simulink model "Optimized_Architecture"  (R2015b)
settings: Solver=FixedStepDiscrete  SolverMode=SingleTasking  StartTime=0.0  StopTime=1000e-6  RelTol=1e-3
libraries: shlslibv1 x282
(part 1 of 2)
settings Model: synDspstartup=OK  Creator=smohan21  LastModifiedBy=smohan21
settings DataIOCC: SaveOutput=off  SignalLogging=off  SaveTime=off
settings OptimizationCC: DefaultParameterBehavior=Inlined
settings DebuggingCC: AlgebraicLoopMsg=error  InheritedTsInSrcMsg=none

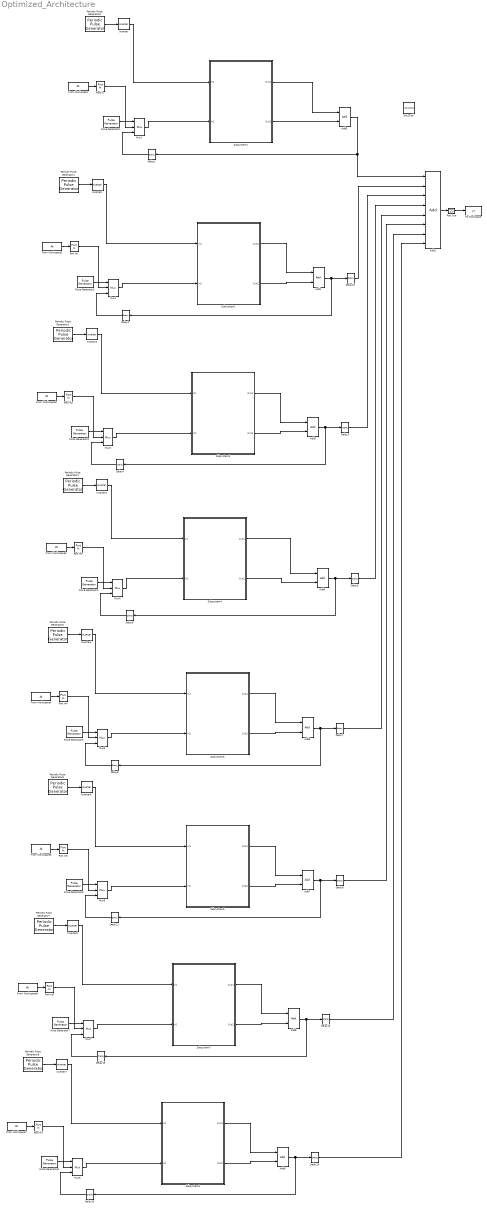
== system Optimized_Architecture ==
  Add{1,3..9} (8 alike) : shlslibv1/Math Functions/Add  syn_add_opr=++  syn_out_f=Specify  syn_out_wl=10  syn_out_fl=0  syn_out_dt=unsigned  syn_out_sat=off  syn_out_rnd=Floor (Truncate)  synBlockType=primitive  synLatency=0  synBlockId=96  syn_sum_of_rows=off  syn_inh_port=off  syn_inh_st=on  syn_inh_stf=1  syn_en_pipe=off  syn_pipe_stg=10  syn_flow_ctrl=off
  Add2 : shlslibv1/Math Functions/Add  syn_add_opr=++++++++  syn_out_f=Specify  syn_out_wl=10  syn_out_fl=0  syn_out_dt=unsigned  syn_out_sat=off  syn_out_rnd=Floor (Truncate)  synBlockType=primitive  synLatency=0  synBlockId=96  syn_sum_of_rows=off  syn_inh_port=off  syn_inh_st=on  syn_inh_stf=1  syn_en_pipe=off  syn_pipe_stg=10  syn_flow_ctrl=off
  Delay{1..2,4,6,8,11,13,15} (8 alike) : shlslibv1/Memories/Delay  syn_delay_val=32  synBlockType=primitive  synLatency=32  synBlockId=104
  Delay10 : shlslibv1/Memories/Delay  syn_delay_val=30  synBlockType=primitive  synLatency=30  synBlockId=104
  Delay12 : shlslibv1/Memories/Delay  syn_delay_val=180  synBlockType=primitive  synLatency=180  synBlockId=104
  Delay14 : shlslibv1/Memories/Delay  syn_delay_val=210  synBlockType=primitive  synLatency=210  synBlockId=104
  Delay3 : shlslibv1/Memories/Delay  syn_delay_val=60  synBlockType=primitive  synLatency=60  synBlockId=104
  Delay5 : shlslibv1/Memories/Delay  syn_delay_val=90  synBlockType=primitive  synLatency=90  synBlockId=104
  Delay7 : shlslibv1/Memories/Delay  syn_delay_val=120  synBlockType=primitive  synLatency=120  synBlockId=104
  Delay9 : shlslibv1/Memories/Delay  syn_delay_val=150  synBlockType=primitive  synLatency=150  synBlockId=104
  From Workspace{,1..7} (8 alike) : FromWorkspace  VariableName=At
  Inverter{,1..7} (8 alike) : shlslibv1/Math Functions/Inverter  syn_out_f=Automatic  syn_out_wl=16  syn_out_fl=8  syn_out_dt=signed  synBlockType=primitive  synLatency=0  synBlockId=10
  Mux{1..8} (8 alike) : shlslibv1/Signal Operations/Mux  syn_in_nb=2  syn_out_f=Specify  syn_out_wl=10  syn_out_fl=0  syn_out_dt=unsigned  syn_en_se=off  synBlockType=primitive  synLatency=0  synBlockId=16
  Periodic Pulse Generator{1..8} (8 alike) : shlslibv1/Sources/Periodic Pulse  Generator  syn_period_type=Constant  syn_period=312  syn_pw_type=Constant  syn_pw=31  syn_pd_type=Constant  syn_pd=0  syn_en_port=off  syn_st=1/1e6  synBlockType=custom  synLatency=0
  Port In{,1..7} (8 alike) : shlslibv1/Ports & Subsystems/Port In  syn_out_wl=10  syn_out_fl=0  syn_out_dt=signed  syn_out_st=-1  syn_capture=off  syn_register=on  syn_out_sat=off  syn_out_rnd=on  synBlockType=port  synLatency=1  synBlockId=0
  Port Out : shlslibv1/Ports & Subsystems/Port Out  syn_capture=off  syn_register=on  synBlockType=port  synLatency=1  synBlockId=1
  Pulse Generator{1..8} (8 alike) : shlslibv1/Sources/Pulse Generator  syn_siggentype=Step (0 to 1)  syn_usectl=off  syn_trigedge=rising  syn_triginit=low  syn_stpdel=31  syn_impwidth=1  syn_impdel=1  syn_st=1/1e6  synBlockType=custom  synLatency=0
  SHLSTool : shlslibv1/SHLSTool  synBlockType=tool  syn_dsp_mode=FPGA
  Subsystem1 : Subsystem
  Subsystem2 : Subsystem
  Subsystem3 : Subsystem
  Subsystem4 : Subsystem
  Subsystem5 : Subsystem
  Subsystem6 : Subsystem
  Subsystem7 : Subsystem
  Subsystem8 : Subsystem
  To Workspace : ToWorkspace  VariableName=yt  SaveFormat=Structure With Time  SampleTime=-1
  wires:
  From Workspace/1 -> Port In/1
  Add5/1 -> Delay1/1, Add2/1
  Periodic Pulse Generator3/1 -> Inverter/1
  Pulse Generator1/1 -> Mux2/1
  Port In/1 -> Mux2/2
  Delay1/1 -> Mux2/3
  Add1/1 -> Delay2/1, Delay10/1
  Delay10/1 -> Add2/2
  Add2/1 -> Port Out/1
  Inverter/1 -> Subsystem2/1(In1)
  Mux2/1 -> Subsystem2/2(In2)
  Subsystem2/1(Out1) -> Add5/1
  Subsystem2/2(Out2) -> Add5/2
  From Workspace1/1 -> Port In1/1
  Periodic Pulse Generator1/1 -> Inverter1/1
  Pulse Generator2/1 -> Mux1/1
  Port In1/1 -> Mux1/2
  Delay2/1 -> Mux1/3
  Inverter1/1 -> Subsystem1/1(In1)
  Mux1/1 -> Subsystem1/2(In2)
  Subsystem1/1(Out1) -> Add1/1
  Subsystem1/2(Out2) -> Add1/2
  Add3/1 -> Delay4/1, Delay3/1
  From Workspace2/1 -> Port In2/1
  Periodic Pulse Generator2/1 -> Inverter2/1
  Pulse Generator3/1 -> Mux3/1
  Port In2/1 -> Mux3/2
  Delay4/1 -> Mux3/3
  Inverter2/1 -> Subsystem3/1(In1)
  Mux3/1 -> Subsystem3/2(In2)
  Subsystem3/1(Out1) -> Add3/1
  Subsystem3/2(Out2) -> Add3/2
  Add4/1 -> Delay6/1, Delay5/1
  From Workspace3/1 -> Port In3/1
  Periodic Pulse Generator4/1 -> Inverter3/1
  Pulse Generator4/1 -> Mux4/1
  Port In3/1 -> Mux4/2
  Delay6/1 -> Mux4/3
  Inverter3/1 -> Subsystem4/1(In1)
  Mux4/1 -> Subsystem4/2(In2)
  Subsystem4/1(Out1) -> Add4/1
  Subsystem4/2(Out2) -> Add4/2
  Add6/1 -> Delay8/1, Delay7/1
  From Workspace4/1 -> Port In4/1
  Periodic Pulse Generator5/1 -> Inverter4/1
  Pulse Generator5/1 -> Mux5/1
  Port In4/1 -> Mux5/2
  Delay8/1 -> Mux5/3
  Inverter4/1 -> Subsystem5/1(In1)
  Mux5/1 -> Subsystem5/2(In2)
  Subsystem5/1(Out1) -> Add6/1
  Subsystem5/2(Out2) -> Add6/2
  Add7/1 -> Delay11/1, Delay9/1
  From Workspace5/1 -> Port In5/1
  Periodic Pulse Generator6/1 -> Inverter5/1
  Pulse Generator6/1 -> Mux6/1
  Port In5/1 -> Mux6/2
  Delay11/1 -> Mux6/3
  Inverter5/1 -> Subsystem6/1(In1)
  Mux6/1 -> Subsystem6/2(In2)
  Subsystem6/1(Out1) -> Add7/1
  Subsystem6/2(Out2) -> Add7/2
  Add8/1 -> Delay13/1, Delay12/1
  From Workspace6/1 -> Port In6/1
  Periodic Pulse Generator7/1 -> Inverter6/1
  Pulse Generator7/1 -> Mux7/1
  Port In6/1 -> Mux7/2
  Delay13/1 -> Mux7/3
  Inverter6/1 -> Subsystem7/1(In1)
  Mux7/1 -> Subsystem7/2(In2)
  Subsystem7/1(Out1) -> Add8/1
  Subsystem7/2(Out2) -> Add8/2
  Add9/1 -> Delay15/1, Delay14/1
  From Workspace7/1 -> Port In7/1
  Periodic Pulse Generator8/1 -> Inverter7/1
  Pulse Generator8/1 -> Mux8/1
  Port In7/1 -> Mux8/2
  Delay15/1 -> Mux8/3
  Inverter7/1 -> Subsystem8/1(In1)
  Mux8/1 -> Subsystem8/2(In2)
  Subsystem8/1(Out1) -> Add9/1
  Subsystem8/2(Out2) -> Add9/2
  Delay3/1 -> Add2/3
  Delay5/1 -> Add2/4
  Delay7/1 -> Add2/5
  Delay9/1 -> Add2/6
  Delay12/1 -> Add2/7
  Delay14/1 -> Add2/8
  Port Out/1 -> To Workspace/1

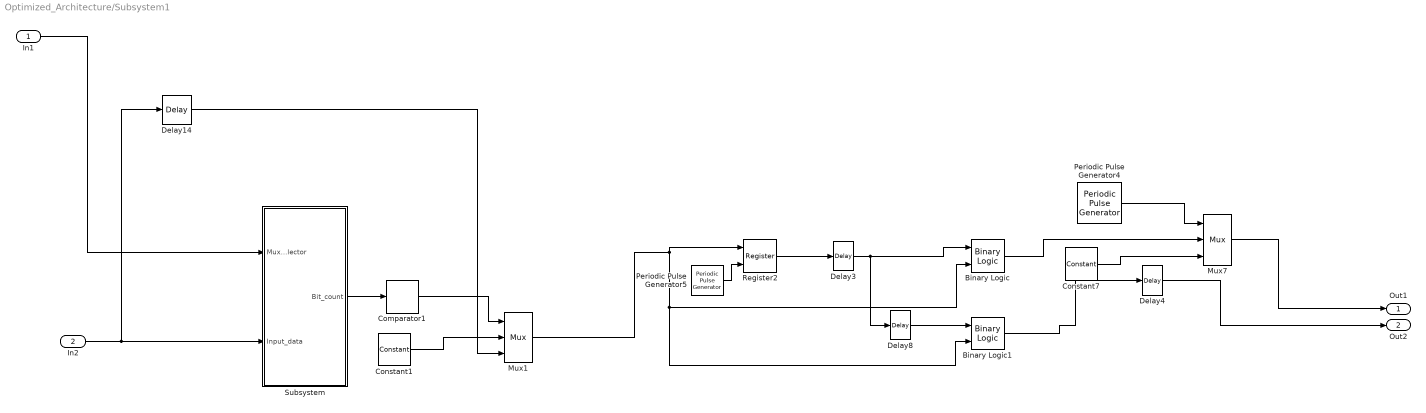
== system Optimized_Architecture/Subsystem1 ==
  In1 : Inport
  In2 : Inport  Port=2
  Binary Logic : shlslibv1/Math Functions/Binary Logic  syn_binlog_exp=a&b  synBlockType=primitive  synLatency=0  synBlockId=13
  Binary Logic1 : shlslibv1/Math Functions/Binary Logic  syn_binlog_exp=a&b  synBlockType=primitive  synLatency=0  synBlockId=13
  Comparator1 : shlslibv1/Math Functions/Comparator  syn_comp_opr=a>=b  syn_comp_const=on  syn_comp_val=2  syn_en_se=off  synBlockType=primitive  synLatency=0  synBlockId=14
  Constant1 : shlslibv1/Sources/Constant  syn_cst_val=0  syn_cst_format=Automatic  syn_cst_wl=1  syn_cst_fl=0  syn_cst_dt=unsigned  syn_cst_rnd=on  syn_cst_st=-1  synBlockType=primitive  synLatency=0  synBlockId=15
  Constant7 : shlslibv1/Sources/Constant  syn_cst_val=0  syn_cst_format=Automatic  syn_cst_wl=1  syn_cst_fl=0  syn_cst_dt=unsigned  syn_cst_rnd=on  syn_cst_st=-1  synBlockType=primitive  synLatency=0  synBlockId=15
  Delay14 : shlslibv1/Memories/Delay  syn_delay_val=270  synBlockType=primitive  synLatency=270  synBlockId=104
  Delay3 : shlslibv1/Memories/Delay  syn_delay_val=9  synBlockType=primitive  synLatency=9  synBlockId=104
  Delay4 : shlslibv1/Memories/Delay  syn_delay_val=10  synBlockType=primitive  synLatency=10  synBlockId=104
  Delay8 : shlslibv1/Memories/Delay  syn_delay_val=10  synBlockType=primitive  synLatency=10  synBlockId=104
  Mux1 : shlslibv1/Signal Operations/Mux  syn_in_nb=2  syn_out_f=Specify  syn_out_wl=10  syn_out_fl=0  syn_out_dt=unsigned  syn_en_se=off  synBlockType=primitive  synLatency=0  synBlockId=16
  Mux7 : shlslibv1/Signal Operations/Mux  syn_in_nb=2  syn_out_f=Specify  syn_out_wl=10  syn_out_fl=0  syn_out_dt=unsigned  syn_en_se=off  synBlockType=primitive  synLatency=0  synBlockId=16
  Periodic Pulse Generator4 : shlslibv1/Sources/Periodic Pulse  Generator  syn_period_type=Constant  syn_period=312  syn_pw_type=Constant  syn_pw=31  syn_pd_type=Constant  syn_pd=0  syn_en_port=off  syn_st=1/1e6  synBlockType=custom  synLatency=0
  Periodic Pulse Generator5 : shlslibv1/Sources/Periodic Pulse  Generator  syn_period_type=Constant  syn_period=270  syn_pw_type=Constant  syn_pw=1  syn_pd_type=Constant  syn_pd=0  syn_en_port=off  syn_st=1/1e6  synBlockType=custom  synLatency=0
  Register2 : shlslibv1/Memories/Register  syn_delay_val=1  syn_rst_val=All zeros  syn_rst_vec=5  syn_rst_port=on  syn_en_port=off  synBlockType=custom  synLatency=1
  Subsystem : Subsystem
  Out1 : Outport
  Out2 : Outport  Port=2
  wires:
  In1/1 -> Subsystem/1(Mux_selector)
  Mux7/1 -> Out1/1
  Mux1/1 -> Register2/1, Binary Logic/2, Binary Logic1/2
  Subsystem/1(Bit_count) -> Comparator1/1
  Constant1/1 -> Mux1/2
  Delay14/1 -> Mux1/3
  Delay3/1 -> Binary Logic/1, Delay8/1
  Binary Logic1/1 -> Delay4/1
  Comparator1/1 -> Mux1/1
  Periodic Pulse Generator4/1 -> Mux7/1
  In2/1 -> Delay14/1, Subsystem/2(Input_data)
  Register2/1 -> Delay3/1
  Delay8/1 -> Binary Logic1/1
  Constant7/1 -> Mux7/3
  Periodic Pulse Generator5/1 -> Register2/2
  Binary Logic/1 -> Mux7/2
  Delay4/1 -> Out2/1

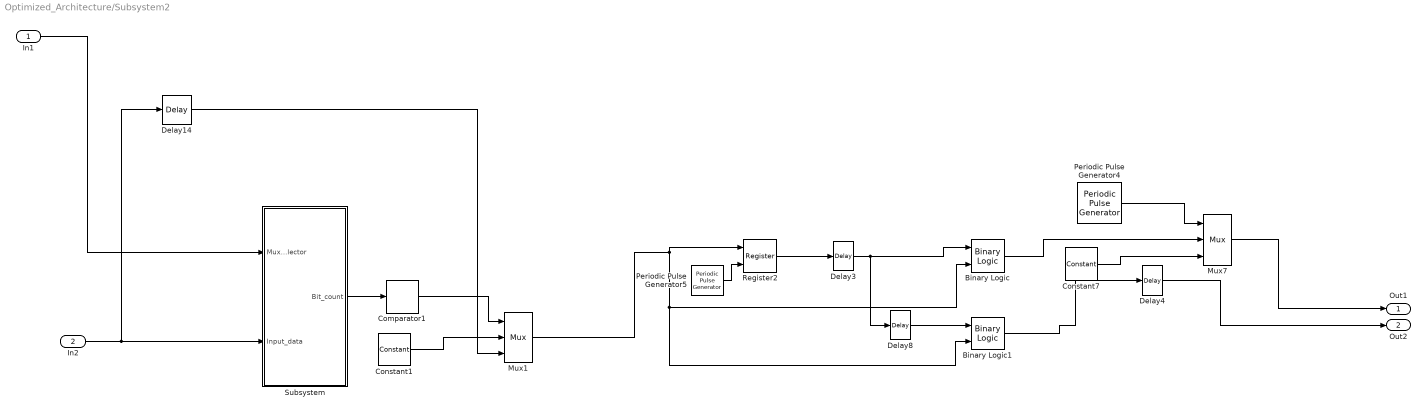
== system Optimized_Architecture/Subsystem2 ==
  In1 : Inport
  In2 : Inport  Port=2
  Binary Logic : shlslibv1/Math Functions/Binary Logic  syn_binlog_exp=a&b  synBlockType=primitive  synLatency=0  synBlockId=13
  Binary Logic1 : shlslibv1/Math Functions/Binary Logic  syn_binlog_exp=a&b  synBlockType=primitive  synLatency=0  synBlockId=13
  Comparator1 : shlslibv1/Math Functions/Comparator  syn_comp_opr=a>=b  syn_comp_const=on  syn_comp_val=2  syn_en_se=off  synBlockType=primitive  synLatency=0  synBlockId=14
  Constant1 : shlslibv1/Sources/Constant  syn_cst_val=0  syn_cst_format=Automatic  syn_cst_wl=1  syn_cst_fl=0  syn_cst_dt=unsigned  syn_cst_rnd=on  syn_cst_st=-1  synBlockType=primitive  synLatency=0  synBlockId=15
  Constant7 : shlslibv1/Sources/Constant  syn_cst_val=0  syn_cst_format=Automatic  syn_cst_wl=1  syn_cst_fl=0  syn_cst_dt=unsigned  syn_cst_rnd=on  syn_cst_st=-1  synBlockType=primitive  synLatency=0  synBlockId=15
  Delay14 : shlslibv1/Memories/Delay  syn_delay_val=270  synBlockType=primitive  synLatency=270  synBlockId=104
  Delay3 : shlslibv1/Memories/Delay  syn_delay_val=9  synBlockType=primitive  synLatency=9  synBlockId=104
  Delay4 : shlslibv1/Memories/Delay  syn_delay_val=10  synBlockType=primitive  synLatency=10  synBlockId=104
  Delay8 : shlslibv1/Memories/Delay  syn_delay_val=10  synBlockType=primitive  synLatency=10  synBlockId=104
  Mux1 : shlslibv1/Signal Operations/Mux  syn_in_nb=2  syn_out_f=Specify  syn_out_wl=10  syn_out_fl=0  syn_out_dt=unsigned  syn_en_se=off  synBlockType=primitive  synLatency=0  synBlockId=16
  Mux7 : shlslibv1/Signal Operations/Mux  syn_in_nb=2  syn_out_f=Specify  syn_out_wl=10  syn_out_fl=0  syn_out_dt=unsigned  syn_en_se=off  synBlockType=primitive  synLatency=0  synBlockId=16
  Periodic Pulse Generator4 : shlslibv1/Sources/Periodic Pulse  Generator  syn_period_type=Constant  syn_period=312  syn_pw_type=Constant  syn_pw=31  syn_pd_type=Constant  syn_pd=0  syn_en_port=off  syn_st=1/1e6  synBlockType=custom  synLatency=0
  Periodic Pulse Generator5 : shlslibv1/Sources/Periodic Pulse  Generator  syn_period_type=Constant  syn_period=270  syn_pw_type=Constant  syn_pw=1  syn_pd_type=Constant  syn_pd=0  syn_en_port=off  syn_st=1/1e6  synBlockType=custom  synLatency=0
  Register2 : shlslibv1/Memories/Register  syn_delay_val=1  syn_rst_val=All zeros  syn_rst_vec=5  syn_rst_port=on  syn_en_port=off  synBlockType=custom  synLatency=1
  Subsystem : Subsystem
  Out1 : Outport
  Out2 : Outport  Port=2
  wires:
  In1/1 -> Subsystem/1(Mux_selector)
  Mux7/1 -> Out1/1
  Mux1/1 -> Register2/1, Binary Logic/2, Binary Logic1/2
  Subsystem/1(Bit_count) -> Comparator1/1
  Constant1/1 -> Mux1/2
  Delay14/1 -> Mux1/3
  Delay3/1 -> Binary Logic/1, Delay8/1
  Binary Logic1/1 -> Delay4/1
  Comparator1/1 -> Mux1/1
  Periodic Pulse Generator4/1 -> Mux7/1
  In2/1 -> Delay14/1, Subsystem/2(Input_data)
  Register2/1 -> Delay3/1
  Delay8/1 -> Binary Logic1/1
  Constant7/1 -> Mux7/3
  Periodic Pulse Generator5/1 -> Register2/2
  Binary Logic/1 -> Mux7/2
  Delay4/1 -> Out2/1

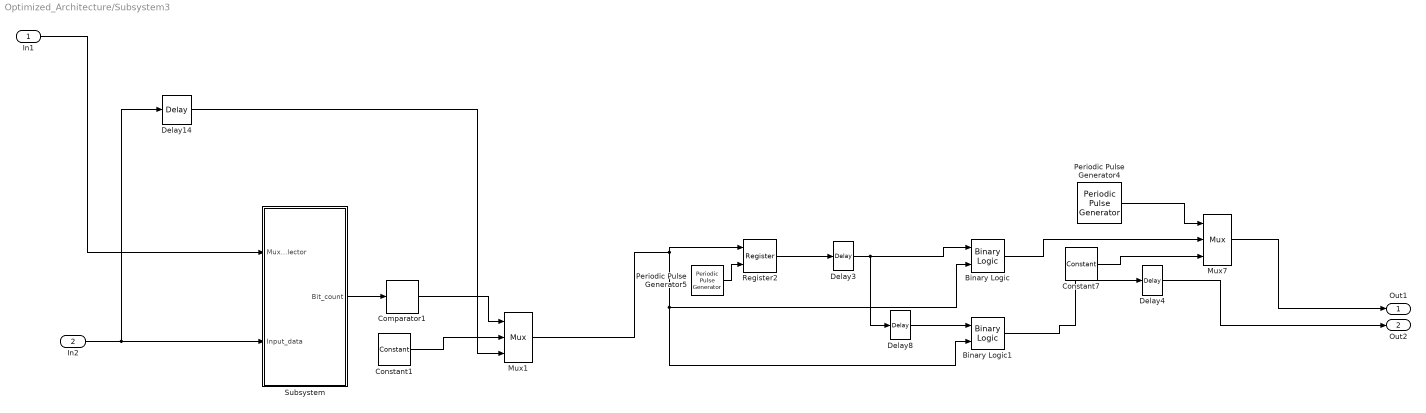
== system Optimized_Architecture/Subsystem3 ==
  In1 : Inport
  In2 : Inport  Port=2
  Binary Logic : shlslibv1/Math Functions/Binary Logic  syn_binlog_exp=a&b  synBlockType=primitive  synLatency=0  synBlockId=13
  Binary Logic1 : shlslibv1/Math Functions/Binary Logic  syn_binlog_exp=a&b  synBlockType=primitive  synLatency=0  synBlockId=13
  Comparator1 : shlslibv1/Math Functions/Comparator  syn_comp_opr=a>=b  syn_comp_const=on  syn_comp_val=2  syn_en_se=off  synBlockType=primitive  synLatency=0  synBlockId=14
  Constant1 : shlslibv1/Sources/Constant  syn_cst_val=0  syn_cst_format=Automatic  syn_cst_wl=1  syn_cst_fl=0  syn_cst_dt=unsigned  syn_cst_rnd=on  syn_cst_st=-1  synBlockType=primitive  synLatency=0  synBlockId=15
  Constant7 : shlslibv1/Sources/Constant  syn_cst_val=0  syn_cst_format=Automatic  syn_cst_wl=1  syn_cst_fl=0  syn_cst_dt=unsigned  syn_cst_rnd=on  syn_cst_st=-1  synBlockType=primitive  synLatency=0  synBlockId=15
  Delay14 : shlslibv1/Memories/Delay  syn_delay_val=270  synBlockType=primitive  synLatency=270  synBlockId=104
  Delay3 : shlslibv1/Memories/Delay  syn_delay_val=9  synBlockType=primitive  synLatency=9  synBlockId=104
  Delay4 : shlslibv1/Memories/Delay  syn_delay_val=10  synBlockType=primitive  synLatency=10  synBlockId=104
  Delay8 : shlslibv1/Memories/Delay  syn_delay_val=10  synBlockType=primitive  synLatency=10  synBlockId=104
  Mux1 : shlslibv1/Signal Operations/Mux  syn_in_nb=2  syn_out_f=Specify  syn_out_wl=10  syn_out_fl=0  syn_out_dt=unsigned  syn_en_se=off  synBlockType=primitive  synLatency=0  synBlockId=16
  Mux7 : shlslibv1/Signal Operations/Mux  syn_in_nb=2  syn_out_f=Specify  syn_out_wl=10  syn_out_fl=0  syn_out_dt=unsigned  syn_en_se=off  synBlockType=primitive  synLatency=0  synBlockId=16
  Periodic Pulse Generator4 : shlslibv1/Sources/Periodic Pulse  Generator  syn_period_type=Constant  syn_period=312  syn_pw_type=Constant  syn_pw=31  syn_pd_type=Constant  syn_pd=0  syn_en_port=off  syn_st=1/1e6  synBlockType=custom  synLatency=0
  Periodic Pulse Generator5 : shlslibv1/Sources/Periodic Pulse  Generator  syn_period_type=Constant  syn_period=270  syn_pw_type=Constant  syn_pw=1  syn_pd_type=Constant  syn_pd=0  syn_en_port=off  syn_st=1/1e6  synBlockType=custom  synLatency=0
  Register2 : shlslibv1/Memories/Register  syn_delay_val=1  syn_rst_val=All zeros  syn_rst_vec=5  syn_rst_port=on  syn_en_port=off  synBlockType=custom  synLatency=1
  Subsystem : Subsystem
  Out1 : Outport
  Out2 : Outport  Port=2
  wires:
  In1/1 -> Subsystem/1(Mux_selector)
  Mux7/1 -> Out1/1
  Mux1/1 -> Register2/1, Binary Logic/2, Binary Logic1/2
  Subsystem/1(Bit_count) -> Comparator1/1
  Constant1/1 -> Mux1/2
  Delay14/1 -> Mux1/3
  Delay3/1 -> Binary Logic/1, Delay8/1
  Binary Logic1/1 -> Delay4/1
  Comparator1/1 -> Mux1/1
  Periodic Pulse Generator4/1 -> Mux7/1
  In2/1 -> Delay14/1, Subsystem/2(Input_data)
  Register2/1 -> Delay3/1
  Delay8/1 -> Binary Logic1/1
  Constant7/1 -> Mux7/3
  Periodic Pulse Generator5/1 -> Register2/2
  Binary Logic/1 -> Mux7/2
  Delay4/1 -> Out2/1

== system Optimized_Architecture/Subsystem4 ==
  In1 : Inport
  In2 : Inport  Port=2
  Binary Logic : shlslibv1/Math Functions/Binary Logic  syn_binlog_exp=a&b  synBlockType=primitive  synLatency=0  synBlockId=13
  Binary Logic1 : shlslibv1/Math Functions/Binary Logic  syn_binlog_exp=a&b  synBlockType=primitive  synLatency=0  synBlockId=13
  Comparator1 : shlslibv1/Math Functions/Comparator  syn_comp_opr=a>=b  syn_comp_const=on  syn_comp_val=2  syn_en_se=off  synBlockType=primitive  synLatency=0  synBlockId=14
  Constant1 : shlslibv1/Sources/Constant  syn_cst_val=0  syn_cst_format=Automatic  syn_cst_wl=1  syn_cst_fl=0  syn_cst_dt=unsigned  syn_cst_rnd=on  syn_cst_st=-1  synBlockType=primitive  synLatency=0  synBlockId=15
  Constant7 : shlslibv1/Sources/Constant  syn_cst_val=0  syn_cst_format=Automatic  syn_cst_wl=1  syn_cst_fl=0  syn_cst_dt=unsigned  syn_cst_rnd=on  syn_cst_st=-1  synBlockType=primitive  synLatency=0  synBlockId=15
  Delay14 : shlslibv1/Memories/Delay  syn_delay_val=270  synBlockType=primitive  synLatency=270  synBlockId=104
  Delay3 : shlslibv1/Memories/Delay  syn_delay_val=9  synBlockType=primitive  synLatency=9  synBlockId=104
  Delay4 : shlslibv1/Memories/Delay  syn_delay_val=10  synBlockType=primitive  synLatency=10  synBlockId=104
  Delay8 : shlslibv1/Memories/Delay  syn_delay_val=10  synBlockType=primitive  synLatency=10  synBlockId=104
  Mux1 : shlslibv1/Signal Operations/Mux  syn_in_nb=2  syn_out_f=Specify  syn_out_wl=10  syn_out_fl=0  syn_out_dt=unsigned  syn_en_se=off  synBlockType=primitive  synLatency=0  synBlockId=16
  Mux7 : shlslibv1/Signal Operations/Mux  syn_in_nb=2  syn_out_f=Specify  syn_out_wl=10  syn_out_fl=0  syn_out_dt=unsigned  syn_en_se=off  synBlockType=primitive  synLatency=0  synBlockId=16
  Periodic Pulse Generator4 : shlslibv1/Sources/Periodic Pulse  Generator  syn_period_type=Constant  syn_period=312  syn_pw_type=Constant  syn_pw=31  syn_pd_type=Constant  syn_pd=0  syn_en_port=off  syn_st=1/1e6  synBlockType=custom  synLatency=0
  Periodic Pulse Generator5 : shlslibv1/Sources/Periodic Pulse  Generator  syn_period_type=Constant  syn_period=270  syn_pw_type=Constant  syn_pw=1  syn_pd_type=Constant  syn_pd=0  syn_en_port=off  syn_st=1/1e6  synBlockType=custom  synLatency=0
  Register2 : shlslibv1/Memories/Register  syn_delay_val=1  syn_rst_val=All zeros  syn_rst_vec=5  syn_rst_port=on  syn_en_port=off  synBlockType=custom  synLatency=1
  Subsystem : Subsystem
  Out1 : Outport
  Out2 : Outport  Port=2
  wires:
  In1/1 -> Subsystem/1(Mux_selector)
  Mux7/1 -> Out1/1
  Mux1/1 -> Register2/1, Binary Logic/2, Binary Logic1/2
  Subsystem/1(Bit_count) -> Comparator1/1
  Constant1/1 -> Mux1/2
  Delay14/1 -> Mux1/3
  Delay3/1 -> Binary Logic/1, Delay8/1
  Binary Logic1/1 -> Delay4/1
  Comparator1/1 -> Mux1/1
  Periodic Pulse Generator4/1 -> Mux7/1
  In2/1 -> Delay14/1, Subsystem/2(Input_data)
  Register2/1 -> Delay3/1
  Delay8/1 -> Binary Logic1/1
  Constant7/1 -> Mux7/3
  Periodic Pulse Generator5/1 -> Register2/2
  Binary Logic/1 -> Mux7/2
  Delay4/1 -> Out2/1

== system Optimized_Architecture/Subsystem5 ==
  In1 : Inport
  In2 : Inport  Port=2
  Binary Logic : shlslibv1/Math Functions/Binary Logic  syn_binlog_exp=a&b  synBlockType=primitive  synLatency=0  synBlockId=13
  Binary Logic1 : shlslibv1/Math Functions/Binary Logic  syn_binlog_exp=a&b  synBlockType=primitive  synLatency=0  synBlockId=13
  Comparator1 : shlslibv1/Math Functions/Comparator  syn_comp_opr=a>=b  syn_comp_const=on  syn_comp_val=2  syn_en_se=off  synBlockType=primitive  synLatency=0  synBlockId=14
  Constant1 : shlslibv1/Sources/Constant  syn_cst_val=0  syn_cst_format=Automatic  syn_cst_wl=1  syn_cst_fl=0  syn_cst_dt=unsigned  syn_cst_rnd=on  syn_cst_st=-1  synBlockType=primitive  synLatency=0  synBlockId=15
  Constant7 : shlslibv1/Sources/Constant  syn_cst_val=0  syn_cst_format=Automatic  syn_cst_wl=1  syn_cst_fl=0  syn_cst_dt=unsigned  syn_cst_rnd=on  syn_cst_st=-1  synBlockType=primitive  synLatency=0  synBlockId=15
  Delay14 : shlslibv1/Memories/Delay  syn_delay_val=270  synBlockType=primitive  synLatency=270  synBlockId=104
  Delay3 : shlslibv1/Memories/Delay  syn_delay_val=9  synBlockType=primitive  synLatency=9  synBlockId=104
  Delay4 : shlslibv1/Memories/Delay  syn_delay_val=10  synBlockType=primitive  synLatency=10  synBlockId=104
  Delay8 : shlslibv1/Memories/Delay  syn_delay_val=10  synBlockType=primitive  synLatency=10  synBlockId=104
  Mux1 : shlslibv1/Signal Operations/Mux  syn_in_nb=2  syn_out_f=Specify  syn_out_wl=10  syn_out_fl=0  syn_out_dt=unsigned  syn_en_se=off  synBlockType=primitive  synLatency=0  synBlockId=16
  Mux7 : shlslibv1/Signal Operations/Mux  syn_in_nb=2  syn_out_f=Specify  syn_out_wl=10  syn_out_fl=0  syn_out_dt=unsigned  syn_en_se=off  synBlockType=primitive  synLatency=0  synBlockId=16
  Periodic Pulse Generator4 : shlslibv1/Sources/Periodic Pulse  Generator  syn_period_type=Constant  syn_period=312  syn_pw_type=Constant  syn_pw=31  syn_pd_type=Constant  syn_pd=0  syn_en_port=off  syn_st=1/1e6  synBlockType=custom  synLatency=0
  Periodic Pulse Generator5 : shlslibv1/Sources/Periodic Pulse  Generator  syn_period_type=Constant  syn_period=270  syn_pw_type=Constant  syn_pw=1  syn_pd_type=Constant  syn_pd=0  syn_en_port=off  syn_st=1/1e6  synBlockType=custom  synLatency=0
  Register2 : shlslibv1/Memories/Register  syn_delay_val=1  syn_rst_val=All zeros  syn_rst_vec=5  syn_rst_port=on  syn_en_port=off  synBlockType=custom  synLatency=1
  Subsystem : Subsystem
  Out1 : Outport
  Out2 : Outport  Port=2
  wires:
  In1/1 -> Subsystem/1(Mux_selector)
  Mux7/1 -> Out1/1
  Mux1/1 -> Register2/1, Binary Logic/2, Binary Logic1/2
  Subsystem/1(Bit_count) -> Comparator1/1
  Constant1/1 -> Mux1/2
  Delay14/1 -> Mux1/3
  Delay3/1 -> Binary Logic/1, Delay8/1
  Binary Logic1/1 -> Delay4/1
  Comparator1/1 -> Mux1/1
  Periodic Pulse Generator4/1 -> Mux7/1
  In2/1 -> Delay14/1, Subsystem/2(Input_data)
  Register2/1 -> Delay3/1
  Delay8/1 -> Binary Logic1/1
  Constant7/1 -> Mux7/3
  Periodic Pulse Generator5/1 -> Register2/2
  Binary Logic/1 -> Mux7/2
  Delay4/1 -> Out2/1

== system Optimized_Architecture/Subsystem6 ==
  In1 : Inport
  In2 : Inport  Port=2
  Binary Logic : shlslibv1/Math Functions/Binary Logic  syn_binlog_exp=a&b  synBlockType=primitive  synLatency=0  synBlockId=13
  Binary Logic1 : shlslibv1/Math Functions/Binary Logic  syn_binlog_exp=a&b  synBlockType=primitive  synLatency=0  synBlockId=13
  Comparator1 : shlslibv1/Math Functions/Comparator  syn_comp_opr=a>=b  syn_comp_const=on  syn_comp_val=2  syn_en_se=off  synBlockType=primitive  synLatency=0  synBlockId=14
  Constant1 : shlslibv1/Sources/Constant  syn_cst_val=0  syn_cst_format=Automatic  syn_cst_wl=1  syn_cst_fl=0  syn_cst_dt=unsigned  syn_cst_rnd=on  syn_cst_st=-1  synBlockType=primitive  synLatency=0  synBlockId=15
  Constant7 : shlslibv1/Sources/Constant  syn_cst_val=0  syn_cst_format=Automatic  syn_cst_wl=1  syn_cst_fl=0  syn_cst_dt=unsigned  syn_cst_rnd=on  syn_cst_st=-1  synBlockType=primitive  synLatency=0  synBlockId=15
  Delay14 : shlslibv1/Memories/Delay  syn_delay_val=270  synBlockType=primitive  synLatency=270  synBlockId=104
  Delay3 : shlslibv1/Memories/Delay  syn_delay_val=9  synBlockType=primitive  synLatency=9  synBlockId=104
  Delay4 : shlslibv1/Memories/Delay  syn_delay_val=10  synBlockType=primitive  synLatency=10  synBlockId=104
  Delay8 : shlslibv1/Memories/Delay  syn_delay_val=10  synBlockType=primitive  synLatency=10  synBlockId=104
  Mux1 : shlslibv1/Signal Operations/Mux  syn_in_nb=2  syn_out_f=Specify  syn_out_wl=10  syn_out_fl=0  syn_out_dt=unsigned  syn_en_se=off  synBlockType=primitive  synLatency=0  synBlockId=16
  Mux7 : shlslibv1/Signal Operations/Mux  syn_in_nb=2  syn_out_f=Specify  syn_out_wl=10  syn_out_fl=0  syn_out_dt=unsigned  syn_en_se=off  synBlockType=primitive  synLatency=0  synBlockId=16
  Periodic Pulse Generator4 : shlslibv1/Sources/Periodic Pulse  Generator  syn_period_type=Constant  syn_period=312  syn_pw_type=Constant  syn_pw=31  syn_pd_type=Constant  syn_pd=0  syn_en_port=off  syn_st=1/1e6  synBlockType=custom  synLatency=0
  Periodic Pulse Generator5 : shlslibv1/Sources/Periodic Pulse  Generator  syn_period_type=Constant  syn_period=270  syn_pw_type=Constant  syn_pw=1  syn_pd_type=Constant  syn_pd=0  syn_en_port=off  syn_st=1/1e6  synBlockType=custom  synLatency=0
  Register2 : shlslibv1/Memories/Register  syn_delay_val=1  syn_rst_val=All zeros  syn_rst_vec=5  syn_rst_port=on  syn_en_port=off  synBlockType=custom  synLatency=1
  Subsystem : Subsystem
  Out1 : Outport
  Out2 : Outport  Port=2
  wires:
  In1/1 -> Subsystem/1(Mux_selector)
  Mux7/1 -> Out1/1
  Mux1/1 -> Register2/1, Binary Logic/2, Binary Logic1/2
  Subsystem/1(Bit_count) -> Comparator1/1
  Constant1/1 -> Mux1/2
  Delay14/1 -> Mux1/3
  Delay3/1 -> Binary Logic/1, Delay8/1
  Binary Logic1/1 -> Delay4/1
  Comparator1/1 -> Mux1/1
  Periodic Pulse Generator4/1 -> Mux7/1
  In2/1 -> Delay14/1, Subsystem/2(Input_data)
  Register2/1 -> Delay3/1
  Delay8/1 -> Binary Logic1/1
  Constant7/1 -> Mux7/3
  Periodic Pulse Generator5/1 -> Register2/2
  Binary Logic/1 -> Mux7/2
  Delay4/1 -> Out2/1

== system Optimized_Architecture/Subsystem7 ==
  In1 : Inport
  In2 : Inport  Port=2
  Binary Logic : shlslibv1/Math Functions/Binary Logic  syn_binlog_exp=a&b  synBlockType=primitive  synLatency=0  synBlockId=13
  Binary Logic1 : shlslibv1/Math Functions/Binary Logic  syn_binlog_exp=a&b  synBlockType=primitive  synLatency=0  synBlockId=13
  Comparator1 : shlslibv1/Math Functions/Comparator  syn_comp_opr=a>=b  syn_comp_const=on  syn_comp_val=2  syn_en_se=off  synBlockType=primitive  synLatency=0  synBlockId=14
  Constant1 : shlslibv1/Sources/Constant  syn_cst_val=0  syn_cst_format=Automatic  syn_cst_wl=1  syn_cst_fl=0  syn_cst_dt=unsigned  syn_cst_rnd=on  syn_cst_st=-1  synBlockType=primitive  synLatency=0  synBlockId=15
  Constant7 : shlslibv1/Sources/Constant  syn_cst_val=0  syn_cst_format=Automatic  syn_cst_wl=1  syn_cst_fl=0  syn_cst_dt=unsigned  syn_cst_rnd=on  syn_cst_st=-1  synBlockType=primitive  synLatency=0  synBlockId=15
  Delay14 : shlslibv1/Memories/Delay  syn_delay_val=270  synBlockType=primitive  synLatency=270  synBlockId=104
  Delay3 : shlslibv1/Memories/Delay  syn_delay_val=9  synBlockType=primitive  synLatency=9  synBlockId=104
  Delay4 : shlslibv1/Memories/Delay  syn_delay_val=10  synBlockType=primitive  synLatency=10  synBlockId=104
  Delay8 : shlslibv1/Memories/Delay  syn_delay_val=10  synBlockType=primitive  synLatency=10  synBlockId=104
  Mux1 : shlslibv1/Signal Operations/Mux  syn_in_nb=2  syn_out_f=Specify  syn_out_wl=10  syn_out_fl=0  syn_out_dt=unsigned  syn_en_se=off  synBlockType=primitive  synLatency=0  synBlockId=16
  Mux7 : shlslibv1/Signal Operations/Mux  syn_in_nb=2  syn_out_f=Specify  syn_out_wl=10  syn_out_fl=0  syn_out_dt=unsigned  syn_en_se=off  synBlockType=primitive  synLatency=0  synBlockId=16
  Periodic Pulse Generator4 : shlslibv1/Sources/Periodic Pulse  Generator  syn_period_type=Constant  syn_period=312  syn_pw_type=Constant  syn_pw=31  syn_pd_type=Constant  syn_pd=0  syn_en_port=off  syn_st=1/1e6  synBlockType=custom  synLatency=0
  Periodic Pulse Generator5 : shlslibv1/Sources/Periodic Pulse  Generator  syn_period_type=Constant  syn_period=270  syn_pw_type=Constant  syn_pw=1  syn_pd_type=Constant  syn_pd=0  syn_en_port=off  syn_st=1/1e6  synBlockType=custom  synLatency=0
  Register2 : shlslibv1/Memories/Register  syn_delay_val=1  syn_rst_val=All zeros  syn_rst_vec=5  syn_rst_port=on  syn_en_port=off  synBlockType=custom  synLatency=1
  Subsystem : Subsystem
  Out1 : Outport
  Out2 : Outport  Port=2
  wires:
  In1/1 -> Subsystem/1(Mux_selector)
  Mux7/1 -> Out1/1
  Mux1/1 -> Register2/1, Binary Logic/2, Binary Logic1/2
  Subsystem/1(Bit_count) -> Comparator1/1
  Constant1/1 -> Mux1/2
  Delay14/1 -> Mux1/3
  Delay3/1 -> Binary Logic/1, Delay8/1
  Binary Logic1/1 -> Delay4/1
  Comparator1/1 -> Mux1/1
  Periodic Pulse Generator4/1 -> Mux7/1
  In2/1 -> Delay14/1, Subsystem/2(Input_data)
  Register2/1 -> Delay3/1
  Delay8/1 -> Binary Logic1/1
  Constant7/1 -> Mux7/3
  Periodic Pulse Generator5/1 -> Register2/2
  Binary Logic/1 -> Mux7/2
  Delay4/1 -> Out2/1

== system Optimized_Architecture/Subsystem8 ==
  In1 : Inport
  In2 : Inport  Port=2
  Binary Logic : shlslibv1/Math Functions/Binary Logic  syn_binlog_exp=a&b  synBlockType=primitive  synLatency=0  synBlockId=13
  Binary Logic1 : shlslibv1/Math Functions/Binary Logic  syn_binlog_exp=a&b  synBlockType=primitive  synLatency=0  synBlockId=13
  Comparator1 : shlslibv1/Math Functions/Comparator  syn_comp_opr=a>=b  syn_comp_const=on  syn_comp_val=2  syn_en_se=off  synBlockType=primitive  synLatency=0  synBlockId=14
  Constant1 : shlslibv1/Sources/Constant  syn_cst_val=0  syn_cst_format=Automatic  syn_cst_wl=1  syn_cst_fl=0  syn_cst_dt=unsigned  syn_cst_rnd=on  syn_cst_st=-1  synBlockType=primitive  synLatency=0  synBlockId=15
  Constant7 : shlslibv1/Sources/Constant  syn_cst_val=0  syn_cst_format=Automatic  syn_cst_wl=1  syn_cst_fl=0  syn_cst_dt=unsigned  syn_cst_rnd=on  syn_cst_st=-1  synBlockType=primitive  synLatency=0  synBlockId=15
  Delay14 : shlslibv1/Memories/Delay  syn_delay_val=270  synBlockType=primitive  synLatency=270  synBlockId=104
  Delay3 : shlslibv1/Memories/Delay  syn_delay_val=9  synBlockType=primitive  synLatency=9  synBlockId=104
  Delay4 : shlslibv1/Memories/Delay  syn_delay_val=10  synBlockType=primitive  synLatency=10  synBlockId=104
  Delay8 : shlslibv1/Memories/Delay  syn_delay_val=10  synBlockType=primitive  synLatency=10  synBlockId=104
  Mux1 : shlslibv1/Signal Operations/Mux  syn_in_nb=2  syn_out_f=Specify  syn_out_wl=10  syn_out_fl=0  syn_out_dt=unsigned  syn_en_se=off  synBlockType=primitive  synLatency=0  synBlockId=16
  Mux7 : shlslibv1/Signal Operations/Mux  syn_in_nb=2  syn_out_f=Specify  syn_out_wl=10  syn_out_fl=0  syn_out_dt=unsigned  syn_en_se=off  synBlockType=primitive  synLatency=0  synBlockId=16
  Periodic Pulse Generator4 : shlslibv1/Sources/Periodic Pulse  Generator  syn_period_type=Constant  syn_period=312  syn_pw_type=Constant  syn_pw=31  syn_pd_type=Constant  syn_pd=0  syn_en_port=off  syn_st=1/1e6  synBlockType=custom  synLatency=0
  Periodic Pulse Generator5 : shlslibv1/Sources/Periodic Pulse  Generator  syn_period_type=Constant  syn_period=270  syn_pw_type=Constant  syn_pw=1  syn_pd_type=Constant  syn_pd=0  syn_en_port=off  syn_st=1/1e6  synBlockType=custom  synLatency=0
  Register2 : shlslibv1/Memories/Register  syn_delay_val=1  syn_rst_val=All zeros  syn_rst_vec=5  syn_rst_port=on  syn_en_port=off  synBlockType=custom  synLatency=1
  Subsystem : Subsystem
  Out1 : Outport
  Out2 : Outport  Port=2
  wires:
  In1/1 -> Subsystem/1(Mux_selector)
  Mux7/1 -> Out1/1
  Mux1/1 -> Register2/1, Binary Logic/2, Binary Logic1/2
  Subsystem/1(Bit_count) -> Comparator1/1
  Constant1/1 -> Mux1/2
  Delay14/1 -> Mux1/3
  Delay3/1 -> Binary Logic/1, Delay8/1
  Binary Logic1/1 -> Delay4/1
  Comparator1/1 -> Mux1/1
  Periodic Pulse Generator4/1 -> Mux7/1
  In2/1 -> Delay14/1, Subsystem/2(Input_data)
  Register2/1 -> Delay3/1
  Delay8/1 -> Binary Logic1/1
  Constant7/1 -> Mux7/3
  Periodic Pulse Generator5/1 -> Register2/2
  Binary Logic/1 -> Mux7/2
  Delay4/1 -> Out2/1

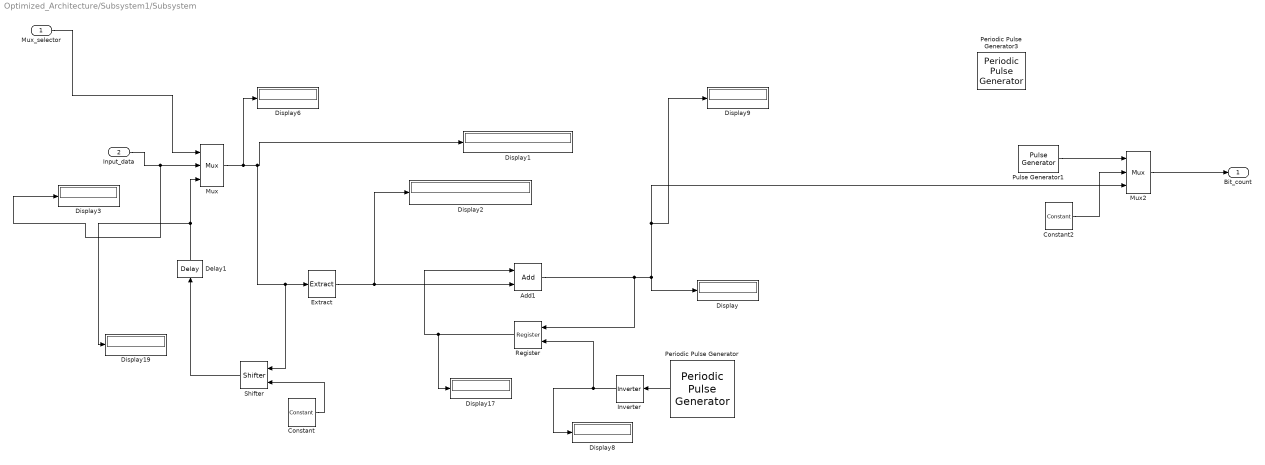
== system Optimized_Architecture/Subsystem1/Subsystem ==
  Mux_selector : Inport
  Input_data : Inport  Port=2
  Add1 : shlslibv1/Math Functions/Add  syn_add_opr=++  syn_out_f=Specify  syn_out_wl=10  syn_out_fl=0  syn_out_dt=unsigned  syn_out_sat=off  syn_out_rnd=Floor (Truncate)  synBlockType=primitive  synLatency=0  synBlockId=96  syn_sum_of_rows=off  syn_inh_port=off  syn_inh_st=on  syn_inh_stf=1  syn_en_pipe=off  syn_pipe_stg=10  syn_flow_ctrl=off
  Constant : shlslibv1/Sources/Constant  syn_cst_val=1  syn_cst_format=Automatic  syn_cst_wl=1  syn_cst_fl=0  syn_cst_dt=unsigned  syn_cst_rnd=on  syn_cst_st=-1  synBlockType=primitive  synLatency=0  synBlockId=15
  Constant2 : shlslibv1/Sources/Constant  syn_cst_val=0  syn_cst_format=Automatic  syn_cst_wl=1  syn_cst_fl=0  syn_cst_dt=unsigned  syn_cst_rnd=on  syn_cst_st=-1  synBlockType=primitive  synLatency=0  synBlockId=15
  Delay1 : shlslibv1/Memories/Delay  syn_delay_val=30  synBlockType=primitive  synLatency=30  synBlockId=104
  Display{,1..3,6,8..9,17,19} (9 alike) : Display
      Display settings: Format=decimal (Stored Integer)
      Display1 settings: Format=binary (Stored Integer)
      Display17 settings: Format=decimal (Stored Integer)
      Display19 settings: Format=decimal (Stored Integer)
      Display2 settings: Format=binary (Stored Integer)
      Display3 settings: Format=decimal (Stored Integer)
      Display8 settings: Format=decimal (Stored Integer)
      Display9 settings: Format=decimal (Stored Integer)
  Extract : shlslibv1/Signal Operations/Extract  syn_extract_vec=0  synBlockType=primitive  synLatency=0  synBlockId=17
  Inverter : shlslibv1/Math Functions/Inverter  syn_out_f=Automatic  syn_out_wl=16  syn_out_fl=8  syn_out_dt=signed  synBlockType=primitive  synLatency=0  synBlockId=10
  Mux : shlslibv1/Signal Operations/Mux  syn_in_nb=2  syn_out_f=Specify  syn_out_wl=10  syn_out_fl=0  syn_out_dt=unsigned  syn_en_se=off  synBlockType=primitive  synLatency=0  synBlockId=16
  Mux2 : shlslibv1/Signal Operations/Mux  syn_in_nb=2  syn_out_f=Specify  syn_out_wl=10  syn_out_fl=0  syn_out_dt=unsigned  syn_en_se=off  synBlockType=primitive  synLatency=0  synBlockId=16
  Periodic Pulse Generator : shlslibv1/Sources/Periodic Pulse  Generator  syn_period_type=Constant  syn_period=309  syn_pw_type=Constant  syn_pw=307  syn_pd_type=Constant  syn_pd=0  syn_en_port=off  syn_st=1/1e6  synBlockType=custom  synLatency=0
  Periodic Pulse Generator3 : shlslibv1/Sources/Periodic Pulse  Generator  syn_period_type=Constant  syn_period=312  syn_pw_type=Constant  syn_pw=31  syn_pd_type=Constant  syn_pd=0  syn_en_port=off  syn_st=1/1e6  synBlockType=custom  synLatency=0
  Pulse Generator1 : shlslibv1/Sources/Pulse Generator  syn_siggentype=Step (0 to 1)  syn_usectl=off  syn_trigedge=rising  syn_triginit=low  syn_stpdel=271  syn_impwidth=1  syn_impdel=1  syn_st=1/1e6  synBlockType=custom  synLatency=0
  Register : shlslibv1/Memories/Register  syn_delay_val=30  syn_rst_val=All zeros  syn_rst_vec=5  syn_rst_port=on  syn_en_port=off  synBlockType=custom  synLatency=30
  Shifter : shlslibv1/Math Functions/Shifter  syn_shifter_opr=>>  syn_out_f=Specify  syn_out_wl=10  syn_out_fl=0  syn_out_dt=unsigned  synBlockType=primitive  synLatency=0  synBlockId=12
  Bit_count : Outport
  wires:
  Add1/1 -> Register/1, Mux2/3, Display9/1, Display/1
  Delay1/1 -> Display19/1, Mux/3
  Constant/1 -> Shifter/2
  Mux_selector/1 -> Mux/1
  Input_data/1 -> Display3/1, Mux/2
  Mux/1 -> Display6/1, Extract/1, Shifter/1, Display1/1
  Periodic Pulse Generator/1 -> Inverter/1
  Register/1 -> Display17/1, Add1/1
  Shifter/1 -> Delay1/1
  Extract/1 -> Display2/1, Add1/2
  Mux2/1 -> Bit_count/1
  Constant2/1 -> Mux2/2
  Inverter/1 -> Register/2, Display8/1
  Pulse Generator1/1 -> Mux2/1

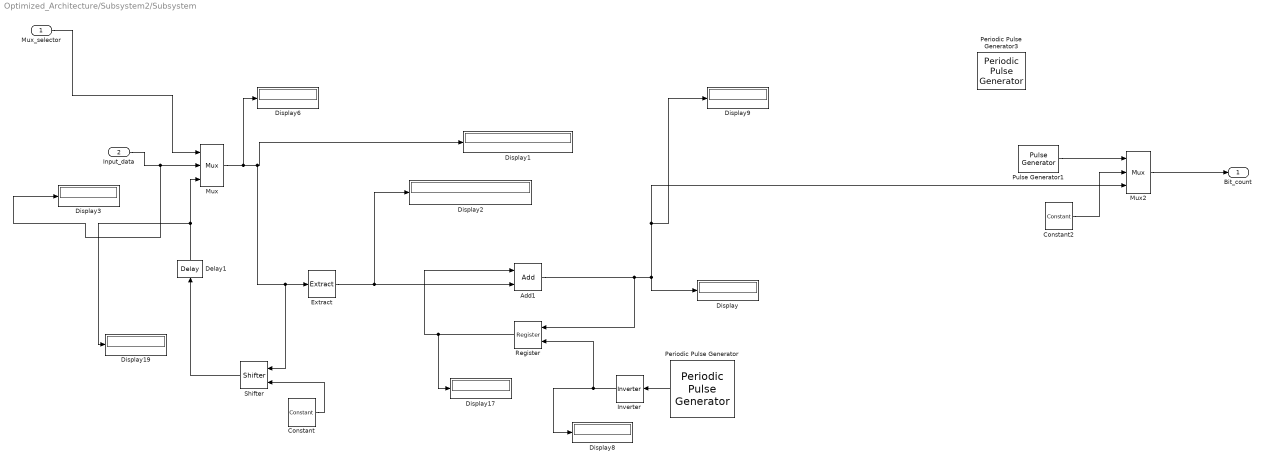
== system Optimized_Architecture/Subsystem2/Subsystem ==
  Mux_selector : Inport
  Input_data : Inport  Port=2
  Add1 : shlslibv1/Math Functions/Add  syn_add_opr=++  syn_out_f=Specify  syn_out_wl=10  syn_out_fl=0  syn_out_dt=unsigned  syn_out_sat=off  syn_out_rnd=Floor (Truncate)  synBlockType=primitive  synLatency=0  synBlockId=96  syn_sum_of_rows=off  syn_inh_port=off  syn_inh_st=on  syn_inh_stf=1  syn_en_pipe=off  syn_pipe_stg=10  syn_flow_ctrl=off
  Constant : shlslibv1/Sources/Constant  syn_cst_val=1  syn_cst_format=Automatic  syn_cst_wl=1  syn_cst_fl=0  syn_cst_dt=unsigned  syn_cst_rnd=on  syn_cst_st=-1  synBlockType=primitive  synLatency=0  synBlockId=15
  Constant2 : shlslibv1/Sources/Constant  syn_cst_val=0  syn_cst_format=Automatic  syn_cst_wl=1  syn_cst_fl=0  syn_cst_dt=unsigned  syn_cst_rnd=on  syn_cst_st=-1  synBlockType=primitive  synLatency=0  synBlockId=15
  Delay1 : shlslibv1/Memories/Delay  syn_delay_val=30  synBlockType=primitive  synLatency=30  synBlockId=104
  Display{,1..3,6,8..9,17,19} (9 alike) : Display
      Display settings: Format=decimal (Stored Integer)
      Display1 settings: Format=binary (Stored Integer)
      Display17 settings: Format=decimal (Stored Integer)
      Display19 settings: Format=decimal (Stored Integer)
      Display2 settings: Format=binary (Stored Integer)
      Display3 settings: Format=decimal (Stored Integer)
      Display8 settings: Format=decimal (Stored Integer)
      Display9 settings: Format=decimal (Stored Integer)
  Extract : shlslibv1/Signal Operations/Extract  syn_extract_vec=0  synBlockType=primitive  synLatency=0  synBlockId=17
  Inverter : shlslibv1/Math Functions/Inverter  syn_out_f=Automatic  syn_out_wl=16  syn_out_fl=8  syn_out_dt=signed  synBlockType=primitive  synLatency=0  synBlockId=10
  Mux : shlslibv1/Signal Operations/Mux  syn_in_nb=2  syn_out_f=Specify  syn_out_wl=10  syn_out_fl=0  syn_out_dt=unsigned  syn_en_se=off  synBlockType=primitive  synLatency=0  synBlockId=16
  Mux2 : shlslibv1/Signal Operations/Mux  syn_in_nb=2  syn_out_f=Specify  syn_out_wl=10  syn_out_fl=0  syn_out_dt=unsigned  syn_en_se=off  synBlockType=primitive  synLatency=0  synBlockId=16
  Periodic Pulse Generator : shlslibv1/Sources/Periodic Pulse  Generator  syn_period_type=Constant  syn_period=309  syn_pw_type=Constant  syn_pw=307  syn_pd_type=Constant  syn_pd=0  syn_en_port=off  syn_st=1/1e6  synBlockType=custom  synLatency=0
  Periodic Pulse Generator3 : shlslibv1/Sources/Periodic Pulse  Generator  syn_period_type=Constant  syn_period=312  syn_pw_type=Constant  syn_pw=31  syn_pd_type=Constant  syn_pd=0  syn_en_port=off  syn_st=1/1e6  synBlockType=custom  synLatency=0
  Pulse Generator1 : shlslibv1/Sources/Pulse Generator  syn_siggentype=Step (0 to 1)  syn_usectl=off  syn_trigedge=rising  syn_triginit=low  syn_stpdel=271  syn_impwidth=1  syn_impdel=1  syn_st=1/1e6  synBlockType=custom  synLatency=0
  Register : shlslibv1/Memories/Register  syn_delay_val=30  syn_rst_val=All zeros  syn_rst_vec=5  syn_rst_port=on  syn_en_port=off  synBlockType=custom  synLatency=30
  Shifter : shlslibv1/Math Functions/Shifter  syn_shifter_opr=>>  syn_out_f=Specify  syn_out_wl=10  syn_out_fl=0  syn_out_dt=unsigned  synBlockType=primitive  synLatency=0  synBlockId=12
  Bit_count : Outport
  wires:
  Add1/1 -> Register/1, Mux2/3, Display9/1, Display/1
  Delay1/1 -> Display19/1, Mux/3
  Constant/1 -> Shifter/2
  Mux_selector/1 -> Mux/1
  Input_data/1 -> Display3/1, Mux/2
  Mux/1 -> Display6/1, Extract/1, Shifter/1, Display1/1
  Periodic Pulse Generator/1 -> Inverter/1
  Register/1 -> Display17/1, Add1/1
  Shifter/1 -> Delay1/1
  Extract/1 -> Display2/1, Add1/2
  Mux2/1 -> Bit_count/1
  Constant2/1 -> Mux2/2
  Inverter/1 -> Register/2, Display8/1
  Pulse Generator1/1 -> Mux2/1

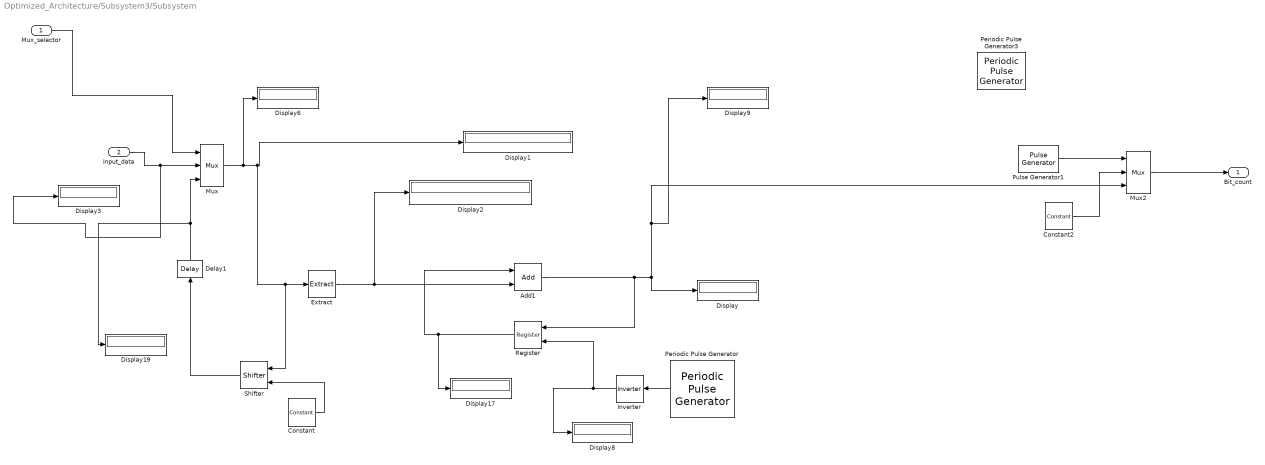
== system Optimized_Architecture/Subsystem3/Subsystem ==
  Mux_selector : Inport
  Input_data : Inport  Port=2
  Add1 : shlslibv1/Math Functions/Add  syn_add_opr=++  syn_out_f=Specify  syn_out_wl=10  syn_out_fl=0  syn_out_dt=unsigned  syn_out_sat=off  syn_out_rnd=Floor (Truncate)  synBlockType=primitive  synLatency=0  synBlockId=96  syn_sum_of_rows=off  syn_inh_port=off  syn_inh_st=on  syn_inh_stf=1  syn_en_pipe=off  syn_pipe_stg=10  syn_flow_ctrl=off
  Constant : shlslibv1/Sources/Constant  syn_cst_val=1  syn_cst_format=Automatic  syn_cst_wl=1  syn_cst_fl=0  syn_cst_dt=unsigned  syn_cst_rnd=on  syn_cst_st=-1  synBlockType=primitive  synLatency=0  synBlockId=15
  Constant2 : shlslibv1/Sources/Constant  syn_cst_val=0  syn_cst_format=Automatic  syn_cst_wl=1  syn_cst_fl=0  syn_cst_dt=unsigned  syn_cst_rnd=on  syn_cst_st=-1  synBlockType=primitive  synLatency=0  synBlockId=15
  Delay1 : shlslibv1/Memories/Delay  syn_delay_val=30  synBlockType=primitive  synLatency=30  synBlockId=104
  Display{,1..3,6,8..9,17,19} (9 alike) : Display
      Display settings: Format=decimal (Stored Integer)
      Display1 settings: Format=binary (Stored Integer)
      Display17 settings: Format=decimal (Stored Integer)
      Display19 settings: Format=decimal (Stored Integer)
      Display2 settings: Format=binary (Stored Integer)
      Display3 settings: Format=decimal (Stored Integer)
      Display8 settings: Format=decimal (Stored Integer)
      Display9 settings: Format=decimal (Stored Integer)
  Extract : shlslibv1/Signal Operations/Extract  syn_extract_vec=0  synBlockType=primitive  synLatency=0  synBlockId=17
  Inverter : shlslibv1/Math Functions/Inverter  syn_out_f=Automatic  syn_out_wl=16  syn_out_fl=8  syn_out_dt=signed  synBlockType=primitive  synLatency=0  synBlockId=10
  Mux : shlslibv1/Signal Operations/Mux  syn_in_nb=2  syn_out_f=Specify  syn_out_wl=10  syn_out_fl=0  syn_out_dt=unsigned  syn_en_se=off  synBlockType=primitive  synLatency=0  synBlockId=16
  Mux2 : shlslibv1/Signal Operations/Mux  syn_in_nb=2  syn_out_f=Specify  syn_out_wl=10  syn_out_fl=0  syn_out_dt=unsigned  syn_en_se=off  synBlockType=primitive  synLatency=0  synBlockId=16
  Periodic Pulse Generator : shlslibv1/Sources/Periodic Pulse  Generator  syn_period_type=Constant  syn_period=309  syn_pw_type=Constant  syn_pw=307  syn_pd_type=Constant  syn_pd=0  syn_en_port=off  syn_st=1/1e6  synBlockType=custom  synLatency=0
  Periodic Pulse Generator3 : shlslibv1/Sources/Periodic Pulse  Generator  syn_period_type=Constant  syn_period=312  syn_pw_type=Constant  syn_pw=31  syn_pd_type=Constant  syn_pd=0  syn_en_port=off  syn_st=1/1e6  synBlockType=custom  synLatency=0
  Pulse Generator1 : shlslibv1/Sources/Pulse Generator  syn_siggentype=Step (0 to 1)  syn_usectl=off  syn_trigedge=rising  syn_triginit=low  syn_stpdel=271  syn_impwidth=1  syn_impdel=1  syn_st=1/1e6  synBlockType=custom  synLatency=0
  Register : shlslibv1/Memories/Register  syn_delay_val=30  syn_rst_val=All zeros  syn_rst_vec=5  syn_rst_port=on  syn_en_port=off  synBlockType=custom  synLatency=30
  Shifter : shlslibv1/Math Functions/Shifter  syn_shifter_opr=>>  syn_out_f=Specify  syn_out_wl=10  syn_out_fl=0  syn_out_dt=unsigned  synBlockType=primitive  synLatency=0  synBlockId=12
  Bit_count : Outport
  wires:
  Add1/1 -> Register/1, Mux2/3, Display9/1, Display/1
  Delay1/1 -> Display19/1, Mux/3
  Constant/1 -> Shifter/2
  Mux_selector/1 -> Mux/1
  Input_data/1 -> Display3/1, Mux/2
  Mux/1 -> Display6/1, Extract/1, Shifter/1, Display1/1
  Periodic Pulse Generator/1 -> Inverter/1
  Register/1 -> Display17/1, Add1/1
  Shifter/1 -> Delay1/1
  Extract/1 -> Display2/1, Add1/2
  Mux2/1 -> Bit_count/1
  Constant2/1 -> Mux2/2
  Inverter/1 -> Register/2, Display8/1
  Pulse Generator1/1 -> Mux2/1

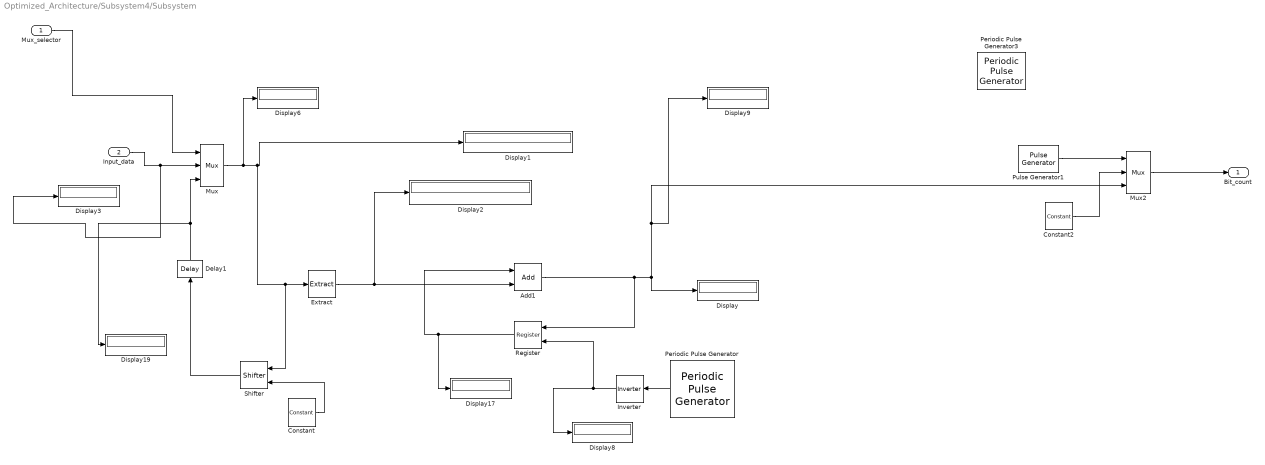
== system Optimized_Architecture/Subsystem4/Subsystem ==
  Mux_selector : Inport
  Input_data : Inport  Port=2
  Add1 : shlslibv1/Math Functions/Add  syn_add_opr=++  syn_out_f=Specify  syn_out_wl=10  syn_out_fl=0  syn_out_dt=unsigned  syn_out_sat=off  syn_out_rnd=Floor (Truncate)  synBlockType=primitive  synLatency=0  synBlockId=96  syn_sum_of_rows=off  syn_inh_port=off  syn_inh_st=on  syn_inh_stf=1  syn_en_pipe=off  syn_pipe_stg=10  syn_flow_ctrl=off
  Constant : shlslibv1/Sources/Constant  syn_cst_val=1  syn_cst_format=Automatic  syn_cst_wl=1  syn_cst_fl=0  syn_cst_dt=unsigned  syn_cst_rnd=on  syn_cst_st=-1  synBlockType=primitive  synLatency=0  synBlockId=15
  Constant2 : shlslibv1/Sources/Constant  syn_cst_val=0  syn_cst_format=Automatic  syn_cst_wl=1  syn_cst_fl=0  syn_cst_dt=unsigned  syn_cst_rnd=on  syn_cst_st=-1  synBlockType=primitive  synLatency=0  synBlockId=15
  Delay1 : shlslibv1/Memories/Delay  syn_delay_val=30  synBlockType=primitive  synLatency=30  synBlockId=104
  Display{,1..3,6,8..9,17,19} (9 alike) : Display
      Display settings: Format=decimal (Stored Integer)
      Display1 settings: Format=binary (Stored Integer)
      Display17 settings: Format=decimal (Stored Integer)
      Display19 settings: Format=decimal (Stored Integer)
      Display2 settings: Format=binary (Stored Integer)
      Display3 settings: Format=decimal (Stored Integer)
      Display8 settings: Format=decimal (Stored Integer)
      Display9 settings: Format=decimal (Stored Integer)
  Extract : shlslibv1/Signal Operations/Extract  syn_extract_vec=0  synBlockType=primitive  synLatency=0  synBlockId=17
  Inverter : shlslibv1/Math Functions/Inverter  syn_out_f=Automatic  syn_out_wl=16  syn_out_fl=8  syn_out_dt=signed  synBlockType=primitive  synLatency=0  synBlockId=10
  Mux : shlslibv1/Signal Operations/Mux  syn_in_nb=2  syn_out_f=Specify  syn_out_wl=10  syn_out_fl=0  syn_out_dt=unsigned  syn_en_se=off  synBlockType=primitive  synLatency=0  synBlockId=16
  Mux2 : shlslibv1/Signal Operations/Mux  syn_in_nb=2  syn_out_f=Specify  syn_out_wl=10  syn_out_fl=0  syn_out_dt=unsigned  syn_en_se=off  synBlockType=primitive  synLatency=0  synBlockId=16
  Periodic Pulse Generator : shlslibv1/Sources/Periodic Pulse  Generator  syn_period_type=Constant  syn_period=309  syn_pw_type=Constant  syn_pw=307  syn_pd_type=Constant  syn_pd=0  syn_en_port=off  syn_st=1/1e6  synBlockType=custom  synLatency=0
  Periodic Pulse Generator3 : shlslibv1/Sources/Periodic Pulse  Generator  syn_period_type=Constant  syn_period=312  syn_pw_type=Constant  syn_pw=31  syn_pd_type=Constant  syn_pd=0  syn_en_port=off  syn_st=1/1e6  synBlockType=custom  synLatency=0
  Pulse Generator1 : shlslibv1/Sources/Pulse Generator  syn_siggentype=Step (0 to 1)  syn_usectl=off  syn_trigedge=rising  syn_triginit=low  syn_stpdel=271  syn_impwidth=1  syn_impdel=1  syn_st=1/1e6  synBlockType=custom  synLatency=0
  Register : shlslibv1/Memories/Register  syn_delay_val=30  syn_rst_val=All zeros  syn_rst_vec=5  syn_rst_port=on  syn_en_port=off  synBlockType=custom  synLatency=30
  Shifter : shlslibv1/Math Functions/Shifter  syn_shifter_opr=>>  syn_out_f=Specify  syn_out_wl=10  syn_out_fl=0  syn_out_dt=unsigned  synBlockType=primitive  synLatency=0  synBlockId=12
  Bit_count : Outport
  wires:
  Add1/1 -> Register/1, Mux2/3, Display9/1, Display/1
  Delay1/1 -> Display19/1, Mux/3
  Constant/1 -> Shifter/2
  Mux_selector/1 -> Mux/1
  Input_data/1 -> Display3/1, Mux/2
  Mux/1 -> Display6/1, Extract/1, Shifter/1, Display1/1
  Periodic Pulse Generator/1 -> Inverter/1
  Register/1 -> Display17/1, Add1/1
  Shifter/1 -> Delay1/1
  Extract/1 -> Display2/1, Add1/2
  Mux2/1 -> Bit_count/1
  Constant2/1 -> Mux2/2
  Inverter/1 -> Register/2, Display8/1
  Pulse Generator1/1 -> Mux2/1

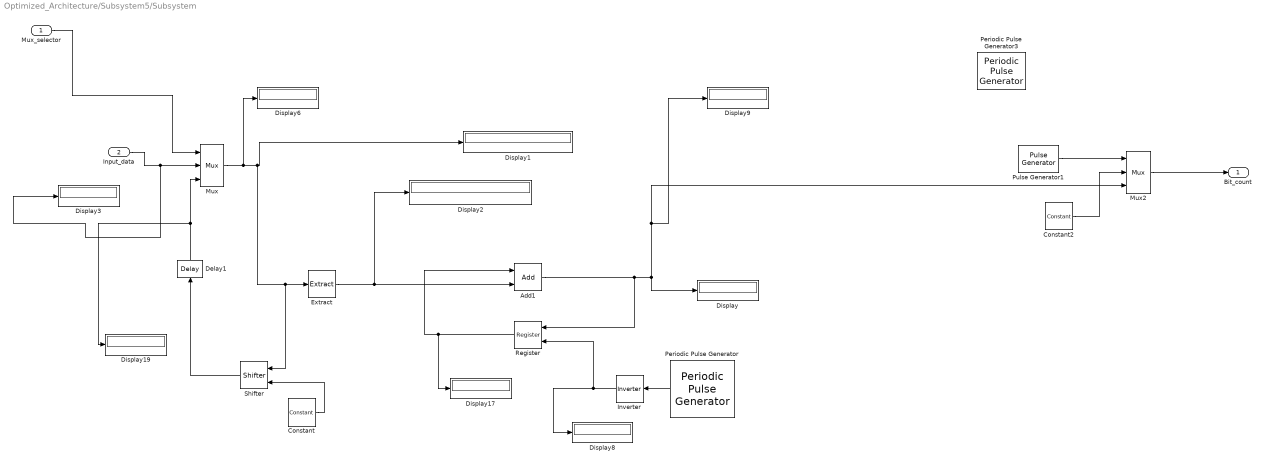
== system Optimized_Architecture/Subsystem5/Subsystem ==
  Mux_selector : Inport
  Input_data : Inport  Port=2
  Add1 : shlslibv1/Math Functions/Add  syn_add_opr=++  syn_out_f=Specify  syn_out_wl=10  syn_out_fl=0  syn_out_dt=unsigned  syn_out_sat=off  syn_out_rnd=Floor (Truncate)  synBlockType=primitive  synLatency=0  synBlockId=96  syn_sum_of_rows=off  syn_inh_port=off  syn_inh_st=on  syn_inh_stf=1  syn_en_pipe=off  syn_pipe_stg=10  syn_flow_ctrl=off
  Constant : shlslibv1/Sources/Constant  syn_cst_val=1  syn_cst_format=Automatic  syn_cst_wl=1  syn_cst_fl=0  syn_cst_dt=unsigned  syn_cst_rnd=on  syn_cst_st=-1  synBlockType=primitive  synLatency=0  synBlockId=15
  Constant2 : shlslibv1/Sources/Constant  syn_cst_val=0  syn_cst_format=Automatic  syn_cst_wl=1  syn_cst_fl=0  syn_cst_dt=unsigned  syn_cst_rnd=on  syn_cst_st=-1  synBlockType=primitive  synLatency=0  synBlockId=15
  Delay1 : shlslibv1/Memories/Delay  syn_delay_val=30  synBlockType=primitive  synLatency=30  synBlockId=104
  Display{,1..3,6,8..9,17,19} (9 alike) : Display
      Display settings: Format=decimal (Stored Integer)
      Display1 settings: Format=binary (Stored Integer)
      Display17 settings: Format=decimal (Stored Integer)
      Display19 settings: Format=decimal (Stored Integer)
      Display2 settings: Format=binary (Stored Integer)
      Display3 settings: Format=decimal (Stored Integer)
      Display8 settings: Format=decimal (Stored Integer)
      Display9 settings: Format=decimal (Stored Integer)
  Extract : shlslibv1/Signal Operations/Extract  syn_extract_vec=0  synBlockType=primitive  synLatency=0  synBlockId=17
  Inverter : shlslibv1/Math Functions/Inverter  syn_out_f=Automatic  syn_out_wl=16  syn_out_fl=8  syn_out_dt=signed  synBlockType=primitive  synLatency=0  synBlockId=10
  Mux : shlslibv1/Signal Operations/Mux  syn_in_nb=2  syn_out_f=Specify  syn_out_wl=10  syn_out_fl=0  syn_out_dt=unsigned  syn_en_se=off  synBlockType=primitive  synLatency=0  synBlockId=16
  Mux2 : shlslibv1/Signal Operations/Mux  syn_in_nb=2  syn_out_f=Specify  syn_out_wl=10  syn_out_fl=0  syn_out_dt=unsigned  syn_en_se=off  synBlockType=primitive  synLatency=0  synBlockId=16
  Periodic Pulse Generator : shlslibv1/Sources/Periodic Pulse  Generator  syn_period_type=Constant  syn_period=309  syn_pw_type=Constant  syn_pw=307  syn_pd_type=Constant  syn_pd=0  syn_en_port=off  syn_st=1/1e6  synBlockType=custom  synLatency=0
  Periodic Pulse Generator3 : shlslibv1/Sources/Periodic Pulse  Generator  syn_period_type=Constant  syn_period=312  syn_pw_type=Constant  syn_pw=31  syn_pd_type=Constant  syn_pd=0  syn_en_port=off  syn_st=1/1e6  synBlockType=custom  synLatency=0
  Pulse Generator1 : shlslibv1/Sources/Pulse Generator  syn_siggentype=Step (0 to 1)  syn_usectl=off  syn_trigedge=rising  syn_triginit=low  syn_stpdel=271  syn_impwidth=1  syn_impdel=1  syn_st=1/1e6  synBlockType=custom  synLatency=0
  Register : shlslibv1/Memories/Register  syn_delay_val=30  syn_rst_val=All zeros  syn_rst_vec=5  syn_rst_port=on  syn_en_port=off  synBlockType=custom  synLatency=30
  Shifter : shlslibv1/Math Functions/Shifter  syn_shifter_opr=>>  syn_out_f=Specify  syn_out_wl=10  syn_out_fl=0  syn_out_dt=unsigned  synBlockType=primitive  synLatency=0  synBlockId=12
  Bit_count : Outport
  wires:
  Add1/1 -> Register/1, Mux2/3, Display9/1, Display/1
  Delay1/1 -> Display19/1, Mux/3
  Constant/1 -> Shifter/2
  Mux_selector/1 -> Mux/1
  Input_data/1 -> Display3/1, Mux/2
  Mux/1 -> Display6/1, Extract/1, Shifter/1, Display1/1
  Periodic Pulse Generator/1 -> Inverter/1
  Register/1 -> Display17/1, Add1/1
  Shifter/1 -> Delay1/1
  Extract/1 -> Display2/1, Add1/2
  Mux2/1 -> Bit_count/1
  Constant2/1 -> Mux2/2
  Inverter/1 -> Register/2, Display8/1
  Pulse Generator1/1 -> Mux2/1
